simulink subsystem "Control"  (R2023a)
settings: Solver=VariableStepAuto  StartTime=0.0  StopTime=10.0  RelTol=1e-3
undefined symbols (not defined in the file or in its folder): arm, nLink
settings Model: Creator=Andy  LastModifiedBy=Andy
settings OptimizationCC: ReuseModelBlockBuffer=off
settings ModelReferenceCC: EnableRefExpFcnMdlSchedulingChecks=on

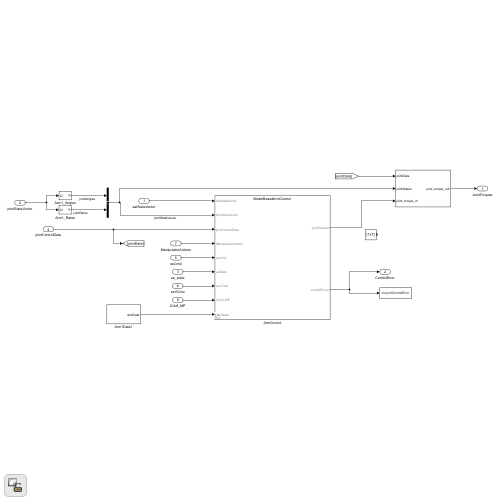
[thumbnail: Simulink's stored preview of the top-level diagram]
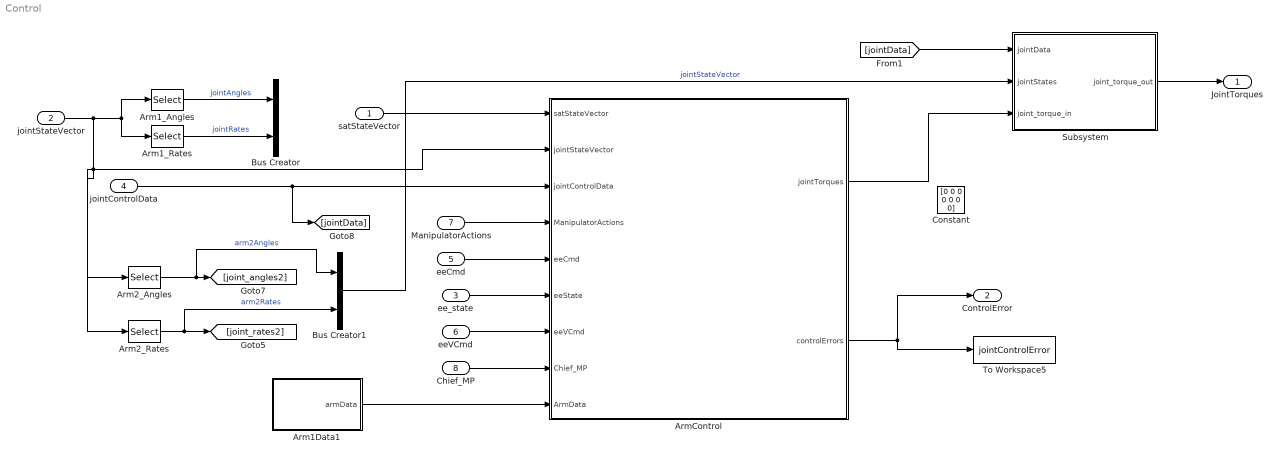
== system Control ==
  satStateVector : Inport
  jointStateVector : Inport  Port=2
  ee_state : Inport  Port=3
  jointControlData : Inport  Port=4
  eeCmd : Inport  Port=5
  eeVCmd : Inport  Port=6
  ManipulatorActions : Inport  Port=7
  Chief_MP : Inport  Port=8
  Arm1Data1 : Subsystem
  Arm1_Angles : Selector  IndexOptions=Index vector (dialog)  Indices=1:arm(1).nLink  OutputSizes=1
  Arm1_Rates : Selector  IndexOptions=Index vector (dialog)  Indices=1+arm(1).nLink+arm(2).nLink:2*arm(1).nLink+arm(2).nLink  OutputSizes=1
  Arm2_Angles : Selector  IndexOptions=Index vector (dialog)  Indices=1+arm(1).nLink:arm(1).nLink+arm(2).nLink  OutputSizes=1
  Arm2_Rates : Selector  IndexOptions=Index vector (dialog)  Indices=1+2*arm(1).nLink+arm(2).nLink:2*arm(1).nLink+2*arm(2).nLink  OutputSizes=1
  ArmControl : Subsystem  Variant=on  VariantControl=Choice
  Bus Creator : BusCreator  Inputs=2
  Bus Creator1 : BusCreator  Inputs=2
  Constant : Constant  Value=[0 0 0 0 0 0 0]
  Subsystem : Subsystem
  To Workspace5 : ToWorkspace  VariableName=jointControlError  SaveFormat=Timeseries  SampleTime=-1
  JointTorques : Outport
  ControlError : Outport  Port=2
  wires:
  jointControlData/1 -> ArmControl/3(jointControlData), [jointData]
  satStateVector/1 -> ArmControl/1(satStateVector)
  ManipulatorActions/1 -> ArmControl/4(ManipulatorActions)
  [jointData] -> Subsystem/1(jointData)
  ArmControl/2(controlErrors) -> To Workspace5/1, ControlError/1
  eeCmd/1 -> ArmControl/5(eeCmd)
  ee_state/1 -> ArmControl/6(eeState)
  eeVCmd/1 -> ArmControl/7(eeVCmd)
  Subsystem/1(joint_torque_out) -> JointTorques/1
  ArmControl/1(jointTorques) -> Subsystem/3(joint_torque_in)
  Chief_MP/1 -> ArmControl/8(Chief_MP)
  Arm1Data1/1(armData) -> ArmControl/9(ArmData)
  Arm1_Angles/1 -> Bus Creator/1  "jointAngles"
  Arm1_Rates/1 -> Bus Creator/2  "jointRates"
  Arm2_Angles/1 -> [joint_angles2], Bus Creator1/1  "arm2Angles"
  Arm2_Rates/1 -> [joint_rates2], Bus Creator1/2  "arm2Rates"
  jointStateVector/1 -> Arm1_Angles/1, Arm1_Rates/1, Arm2_Angles/1, Arm2_Rates/1, ArmControl/2(jointStateVector)
  Bus Creator1/1 -> Subsystem/2(jointStates)  "jointStateVector"

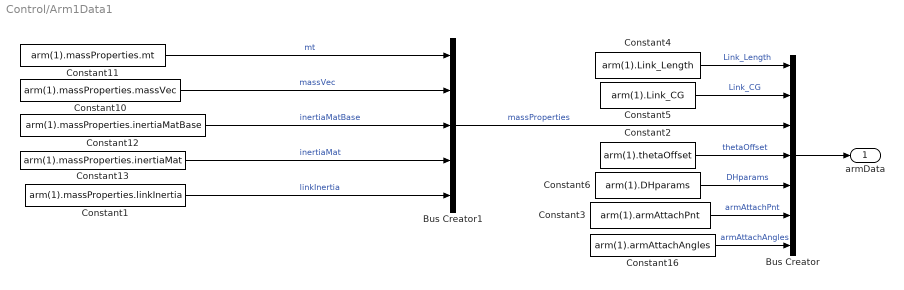
== system Control/Arm1Data1 ==
  Bus Creator : BusCreator  Inputs=7
  Bus Creator1 : BusCreator  Inputs=5  OutDataTypeStr=Bus: MassPropertiesBus
      settings: InheritFromInputs=off
  Constant1 : Constant  Value=arm(1).massProperties.linkInertia
  Constant10 : Constant  Value=arm(1).massProperties.massVec
  Constant11 : Constant  Value=arm(1).massProperties.mt
  Constant12 : Constant  Value=arm(1).massProperties.inertiaMatBase
  Constant13 : Constant  Value=arm(1).massProperties.inertiaMat
  Constant16 : Constant  Value=arm(1).armAttachAngles
  Constant2 : Constant  Value=arm(1).thetaOffset
  Constant3 : Constant  Value=arm(1).armAttachPnt
  Constant4 : Constant  Value=arm(1).Link_Length
  Constant5 : Constant  Value=arm(1).Link_CG
  Constant6 : Constant  Value=arm(1).DHparams
  armData : Outport
  wires:
  Constant1/1 -> Bus Creator1/5  "linkInertia"
  Bus Creator/1 -> armData/1
  Constant16/1 -> Bus Creator/7  "armAttachAngles"
  Constant3/1 -> Bus Creator/6  "armAttachPnt"
  Constant4/1 -> Bus Creator/1  "Link_Length"
  Constant5/1 -> Bus Creator/2  "Link_CG"
  Constant6/1 -> Bus Creator/5  "DHparams"
  Constant2/1 -> Bus Creator/4  "thetaOffset"
  Constant12/1 -> Bus Creator1/3  "inertiaMatBase"
  Constant13/1 -> Bus Creator1/4  "inertiaMat"
  Constant10/1 -> Bus Creator1/2  "massVec"
  Constant11/1 -> Bus Creator1/1  "mt"
  Bus Creator1/1 -> Bus Creator/3  "massProperties"

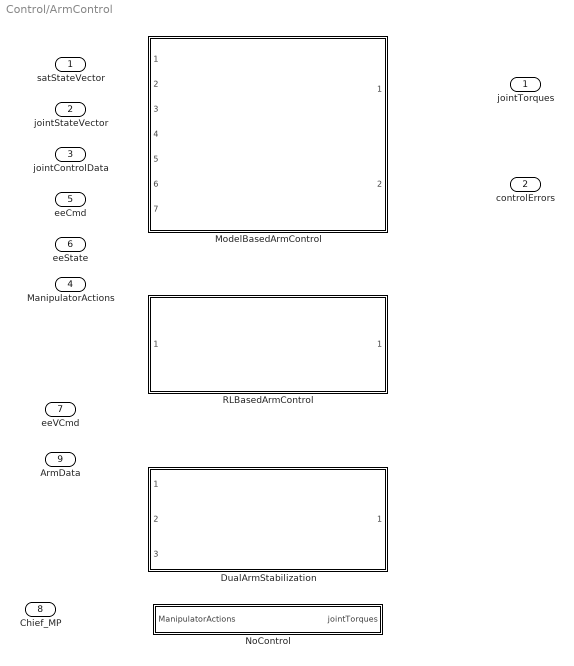
== system Control/ArmControl ==
  satStateVector : Inport
  jointStateVector : Inport  Port=2
  jointControlData : Inport  Port=3
  ManipulatorActions : Inport  Port=4
  eeCmd : Inport  Port=5
  eeState : Inport  Port=6
  eeVCmd : Inport  Port=7
  Chief_MP : Inport  Port=8
  ArmData : Inport  Port=9
  DualArmStabilization : Subsystem  VariantControl=VSS_DualArmStabilization  ReferencedSubsystem=DualArmStabilization
  ModelBasedArmControl : Subsystem  VariantControl=VSS_ModelBasedArmControl  ReferencedSubsystem=ModelBasedArmControl
  NoControl : Subsystem  VariantControl=VSS_NoControl
  RLBasedArmControl : Subsystem  VariantControl=VSS_RLBasedArmControl  ReferencedSubsystem=RLBasedArmControl
  jointTorques : Outport
  controlErrors : Outport  Port=2

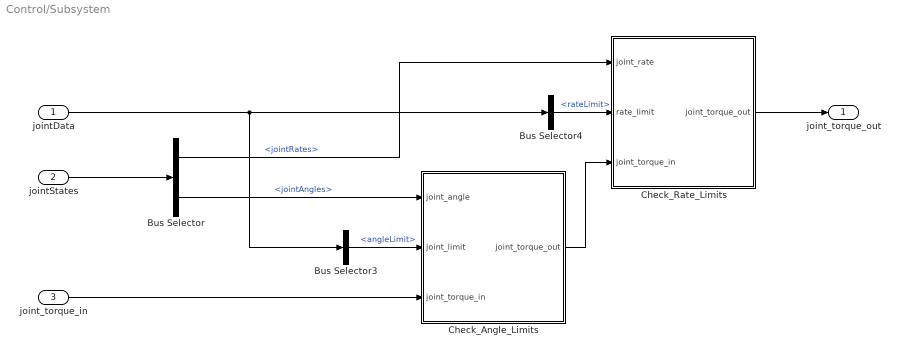
== system Control/Subsystem ==
  jointData : Inport
  jointStates : Inport  Port=2
  joint_torque_in : Inport  Port=3
  Bus Selector : BusSelector  OutputSignals=jointRates,jointAngles
  Bus Selector3 : BusSelector  OutputSignals=angleLimit
  Bus Selector4 : BusSelector  OutputSignals=rateLimit
  Check_Angle_Limits : MATLAB Function
  Check_Rate_Limits : MATLAB Function
  joint_torque_out : Outport
  wires:
  Bus Selector/1 -> Check_Rate_Limits/1(joint_rate)  "<jointRates>"
  jointStates/1 -> Bus Selector/1
  Check_Rate_Limits/1(joint_torque_out) -> joint_torque_out/1
  joint_torque_in/1 -> Check_Angle_Limits/3(joint_torque_in)
  Bus Selector3/1 -> Check_Angle_Limits/2(joint_limit)  "<angleLimit>"
  Check_Angle_Limits/1(joint_torque_out) -> Check_Rate_Limits/3(joint_torque_in)
  Bus Selector4/1 -> Check_Rate_Limits/2(rate_limit)  "<rateLimit>"
  jointData/1 -> Bus Selector4/1, Bus Selector3/1
  Bus Selector/2 -> Check_Angle_Limits/1(joint_angle)  "<jointAngles>"

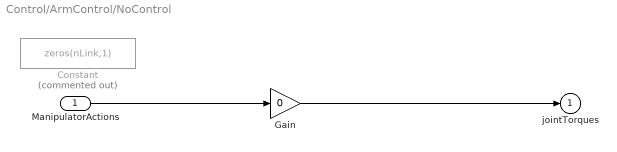
== system Control/ArmControl/NoControl ==
  ManipulatorActions : Inport
  Constant : Constant  Commented=on  Value=zeros(nLink,1)
  Gain : Gain  Gain=0
  jointTorques : Outport
  wires:
  Gain/1 -> jointTorques/1
  ManipulatorActions/1 -> Gain/1

== matlab function Control/Subsystem/Check_Angle_Limits ==
  data: joint_torque_out output; joint_angle input; joint_limit input; joint_torque_in input; NLINKS parameter
function joint_torque_out = Check_Angle_Limits(joint_angle,joint_limit,joint_torque_in,NLINKS)

% The line below broke the signal size back propagation, so instead set
% it to zeros and set each element individually
% joint_torque_out = joint_torque_in; 

joint_torque_out = zeros(NLINKS,1);

% If the current angle is near the limit and the torque continues
% to move that direction, zero it.
for i = 1:NLINKS
    if joint_angle(i) < 0
        % Negative case
        if joint_angle(i)/joint_limit(i,1) > 0.95 && joint_torque_in(i) < 0
            joint_torque_out(i) = 0.0;
        else
            joint_torque_out(i) = joint_torque_in(i);
        end
    else
        % Positive case
        if joint_angle(i)/joint_limit(i,2) > 0.95 && joint_torque_in(i) > 0
            joint_torque_out(i) = 0.0;
        else
            joint_torque_out(i) = joint_torque_in(i);
        end
    end
end

== matlab function Control/Subsystem/Check_Rate_Limits ==
  data: joint_torque_out output; joint_rate input; rate_limit input; joint_torque_in input; NLINKS parameter
function joint_torque_out = Check_Rate_Limits(joint_rate,rate_limit,joint_torque_in,NLINKS)

% The line below broke the signal size back propagation, so instead set
% it to zeros and set each element individually
% joint_torque_out = joint_torque_in; 

joint_torque_out = zeros(NLINKS,1);

% If the current rate is at or above the limit and the torque command would
% continue to move that direction, zero it.

for i = 1:NLINKS
    if joint_rate(i) < 0
        % Negative case
        if abs(joint_rate(i)) >= rate_limit(i) && joint_torque_in(i) < 0
            joint_torque_out(i) = 0.0;
        else
            joint_torque_out(i) = joint_torque_in(i);
        end
    else
        % Positive case
        if abs(joint_rate(i)) >= rate_limit(i) && joint_torque_in(i) > 0
            joint_torque_out(i) = 0.0;
        else
            joint_torque_out(i) = joint_torque_in(i);
        end
    end
end
